simulink model "sampleModel1736"  (R2022a)
settings: Solver=FixedStepAuto  StartTime=0.0  StopTime=10.0  RelTol=1e-3
undefined symbols (not defined in the file): DiscIntNeverNeededParam, magnitude, Newton, Raphson
libraries: simulink x102, slpidlib x27
(part 1 of 4)
settings Model: SimulationMode=software-in-the-loop (sil)  Creator=lenovo  LastModifiedBy=TSMC
settings DataIOCC: InspectSignalLogs=on  SignalLoggingName=logsOut
settings OptimizationCC: DefaultParameterBehavior=Inlined  EnhancedBackFolding=on  PassReuseOutputArgsAs=Individual arguments  ZeroExternalMemoryAtStartup=off  ZeroInternalMemoryAtStartup=off  OptimizeBlockOrder=speed  DifferentSizesBufferReuse=on  OptimizationCustomize=off  EfficientTunableParamExpr=on
settings DebuggingCC: ParameterTunabilityLossMsg=error  UnconnectedInputMsg=warning  UnconnectedOutputMsg=warning  UnconnectedLineMsg=warning
settings ModelReferenceCC: UpdateModelReferenceTargets=Force
settings SFSimCC: MATLABDynamicMemAlloc=off
settings RTWCC: SystemTargetFile=ert.tlc  TemplateMakefile=ert_default_tmf  GenerateReport=on  IncludeHyperlinkInReport=on  GenerateTraceInfo=on  DLArmComputeVersion=19.05
settings CodeAppCC: ForceParamTrailComments=on  IgnoreCustomStorageClasses=off  OperatorAnnotations=on  SimulinkDataObjDesc=on  SFDataObjDesc=on  InsertBlockDesc=on
settings ERTTargetCC: TargetLangStandard=C99 (ISO)  GenerateSampleERTMain=on  SupportContinuousTime=on  InlinedParameterPlacement=NonHierarchical  ERTCustomFileTemplate=example_file_process.tlc

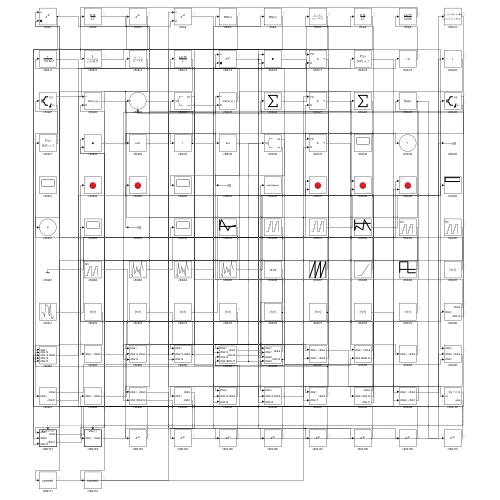
[thumbnail: Simulink's stored preview of the top-level diagram]
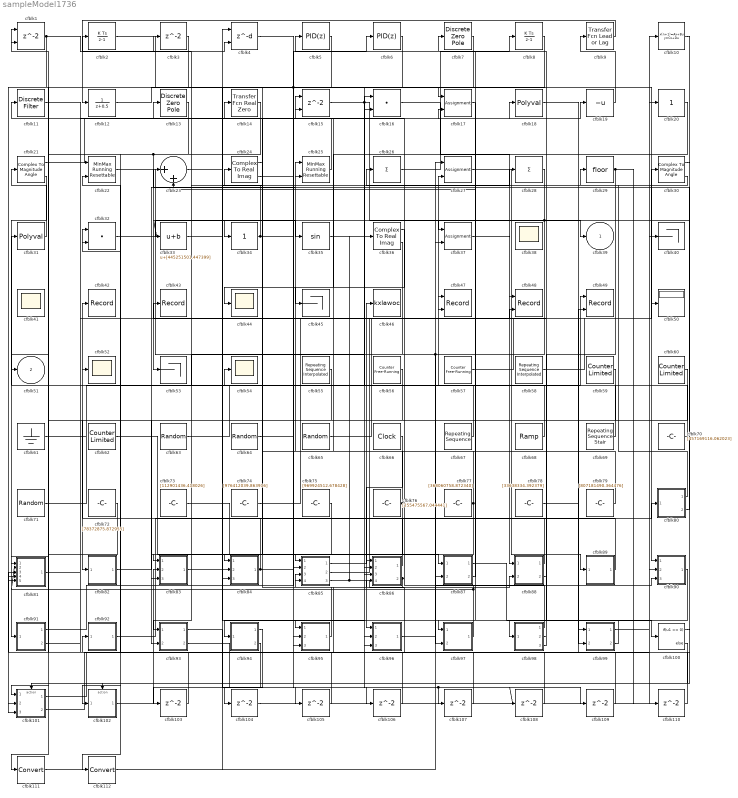
== system sampleModel1736 ==
  cfblk1 : Delay  ShowEnablePort=on  SampleTime=1
      settings: InputPortMap=u0,e6
  cfblk10 : DiscreteStateSpace
  cfblk100 : If  IfExpression=u1 >= 0  SampleTime=1
  cfblk101 : Subsystem  TreatAsAtomicUnit=on
  cfblk102 : Subsystem  TreatAsAtomicUnit=on
  cfblk{3,103..110} (9 alike) : Delay  SampleTime=1
  cfblk11 : DiscreteFilter  SampleTime=1
  cfblk111 : DataTypeConversion  SaturateOnIntegerOverflow=off  RndMeth=Floor
  cfblk112 : DataTypeConversion  SaturateOnIntegerOverflow=off  RndMeth=Floor
  cfblk12 : DiscreteTransferFcn  SampleTime=1
  cfblk13 : DiscreteZeroPole  Poles=[0 0.5]  Gain=1
  cfblk14 : simulink/Discrete/Transfer Fcn Real Zero  ZeroZ=0.75  ICPrevInput=0.0  DoSatur=off
      settings: SourceProductBaseCode=SL
  cfblk15 : Delay  ShowEnablePort=on  SampleTime=1
      settings: InputPortMap=u0,e6
  cfblk16 : DotProduct  OutDataTypeStr=Inherit: Inherit via internal rule
  cfblk17 : Assignment  DiagnosticForDimensions=Warning  IndexOptions=Index vector (dialog)  Indices=1  OutputSizes=1
  cfblk18 : Polyval  Coefs=[ +2.081618890e-019, -1.441693666e-014, +4.719686976e-010, -8.536869453e-006, +1.621573104e-001, -8.087801117e+001 ]
  cfblk19 : UnaryMinus
  cfblk2 : DiscreteIntegrator  ICPrevOutput=DiscIntNeverNeededParam  ICPrevScaledInput=DiscIntNeverNeededParam
  cfblk20 : simulink/Math Operations/Slider Gain  gain=1  low=0  high=2
  cfblk21 : ComplexToMagnitudeAngle
  cfblk22 : simulink/Math Operations/MinMax Running Resettable  Function=min  vinit=0.0
  cfblk23 : Sum  Inputs=|++
  cfblk24 : ComplexToRealImag
  cfblk25 : simulink/Math Operations/MinMax Running Resettable  Function=min  vinit=0.0
  cfblk26 : Sum  Inputs=+
  cfblk27 : Assignment  DiagnosticForDimensions=Warning  IndexOptions=Index vector (dialog)  Indices=1  OutputSizes=1
  cfblk28 : Sum  Inputs=+
  cfblk29 : Rounding
  cfblk30 : ComplexToMagnitudeAngle
  cfblk31 : Polyval  Coefs=[ +2.081618890e-019, -1.441693666e-014, +4.719686976e-010, -8.536869453e-006, +1.621573104e-001, -8.087801117e+001 ]
  cfblk32 : DotProduct  OutDataTypeStr=Inherit: Inherit via internal rule
  cfblk33 : Bias  Bias=[445251501.447399]  SaturateOnIntegerOverflow=off
  cfblk34 : simulink/Math Operations/Slider Gain  gain=1  low=0  high=2
  cfblk35 : Trigonometry
  cfblk36 : ComplexToRealImag
  cfblk37 : Assignment  DiagnosticForDimensions=Warning  IndexOptions=Index vector (dialog)  Indices=1  OutputSizes=1
  cfblk{38,41,44,52,54} (5 alike) : Scope
      cfblk38 settings: Floating=on
      cfblk41 settings: Floating=on
  cfblk4 : Delay  DelayLengthSource=Input port  SampleTime=1
      settings: InputPortMap=u0,p1
  cfblk40 : Terminator
  cfblk42 : Record  FileSettingsInternal="{\"entries\":[{\"content\":{\"excelSettings\":{\"content\":{},\"type\":\"Streamout.ExcelSettings\"}},\"type\":\"Streamout.FileSettingStorage\",\"uuid\":\"672957eb-ee49-4fe5-a35a-1dea1006cdd7\"}],\"packageUris\":[\"http://schema.mathworks.com/mf0/streamout_blocks/R2020a\"],\"version\":\"1.0\"}"  SignalsInternal="{\"entries\":[{\"content\":{\"signals\":[]},\"type\":\"RecordBlkView.InputSignals\",\"uuid\":\"5e46232b-0d34-4261-b03a-cdc6809bb342\"}],\"packageUris\":[\"http://schema.mathworks.com/mf0/streamout_blocks/R2020a\"],\"version\":\"1.0\"}"  VisualizationBindings="{\"sparklinesplugin\":{\"info\":[{\"bindingParametersList\":[],\"subplotID\":1}]}}"
  cfblk43 : Record  FileSettingsInternal="{\"entries\":[{\"content\":{\"excelSettings\":{\"content\":{},\"type\":\"Streamout.ExcelSettings\"}},\"type\":\"Streamout.FileSettingStorage\",\"uuid\":\"393a2e3c-94c8-4af6-8f54-ad1e74355c79\"}],\"packageUris\":[\"http://schema.mathworks.com/mf0/streamout_blocks/R2020a\"],\"version\":\"1.0\"}"  SignalsInternal="{\"entries\":[{\"content\":{\"signals\":[]},\"type\":\"RecordBlkView.InputSignals\",\"uuid\":\"d289a954-6309-4463-a7cf-1981229a1c79\"}],\"packageUris\":[\"http://schema.mathworks.com/mf0/streamout_blocks/R2020a\"],\"version\":\"1.0\"}"  VisualizationBindings="{\"sparklinesplugin\":{\"info\":[{\"bindingParametersList\":[],\"subplotID\":1}]}}"
  cfblk45 : Terminator
  cfblk46 : ToWorkspace  VariableName=kxlawoc  SaveFormat=Timeseries  SampleTime=-1
  cfblk47 : Record  FileSettingsInternal="{\"entries\":[{\"content\":{\"excelSettings\":{\"content\":{},\"type\":\"Streamout.ExcelSettings\"}},\"type\":\"Streamout.FileSettingStorage\",\"uuid\":\"0105e05e-0964-4cfc-9bef-5427dfc10fd6\"}],\"packageUris\":[\"http://schema.mathworks.com/mf0/streamout_blocks/R2020a\"],\"version\":\"1.0\"}"  Layout=[1 1]  SignalsInternal="{\"entries\":[{\"content\":{\"signals\":[]},\"type\":\"RecordBlkView.InputSignals\",\"uuid\":\"b76d1c99-58a2-4a2f-b9d3-63975c932613\"}],\"packageUris\":[\"http://schema.mathworks.com/mf0/streamout_blocks/R2020a\"],\"version\":\"1.0\"}"  VisualizationBindings="{\"xyplotplugin\":{\"info\":[{\"series\":[],\"subplotID\":1}]}}"  CompatibilityTag=XY  st=-1
  cfblk48 : Record  FileSettingsInternal="{\"entries\":[{\"content\":{\"excelSettings\":{\"content\":{},\"type\":\"Streamout.ExcelSettings\"}},\"type\":\"Streamout.FileSettingStorage\",\"uuid\":\"b0e192a8-91e4-4ef8-ad00-b270703470c1\"}],\"packageUris\":[\"http://schema.mathworks.com/mf0/streamout_blocks/R2020a\"],\"version\":\"1.0\"}"  Layout=[1 1]  SignalsInternal="{\"entries\":[{\"content\":{\"signals\":[]},\"type\":\"RecordBlkView.InputSignals\",\"uuid\":\"d4c1af31-3cad-49f8-ac33-698687fb22b3\"}],\"packageUris\":[\"http://schema.mathworks.com/mf0/streamout_blocks/R2020a\"],\"version\":\"1.0\"}"  VisualizationBindings="{\"xyplotplugin\":{\"info\":[{\"series\":[],\"subplotID\":1}]}}"  CompatibilityTag=XY  st=-1
  cfblk49 : Record  FileSettingsInternal="{\"entries\":[{\"content\":{\"excelSettings\":{\"content\":{},\"type\":\"Streamout.ExcelSettings\"}},\"type\":\"Streamout.FileSettingStorage\",\"uuid\":\"edb0e36a-dec4-460e-bf37-95f7f6bcaa08\"}],\"packageUris\":[\"http://schema.mathworks.com/mf0/streamout_blocks/R2020a\"],\"version\":\"1.0\"}"  Layout=[1 1]  SignalsInternal="{\"entries\":[{\"content\":{\"signals\":[]},\"type\":\"RecordBlkView.InputSignals\",\"uuid\":\"dacf59fe-381c-43c7-bd7c-2111ca233486\"}],\"packageUris\":[\"http://schema.mathworks.com/mf0/streamout_blocks/R2020a\"],\"version\":\"1.0\"}"  VisualizationBindings="{\"xyplotplugin\":{\"info\":[{\"series\":[],\"subplotID\":1}]}}"  CompatibilityTag=XY  st=-1
  cfblk5 : slpidlib/PID Controller  Controller=PID  Form=Parallel  TimeDomain=Discrete-time  UseExternalTs=off  SampleTime=1  IntegratorMethod=Forward Euler  FilterMethod=Forward Euler  ControllerParametersSource=internal  P=1  I=1  UseKiTs=off  D=0  N=100  UseFilter=on  TunerSelectOption=Transfer Function Based (PID Tuner App)  InitialConditionSource=internal  InitialConditionForIntegrator=0  InitialConditionForFilter=0  DifferentiatorICPrevScaledInput=0  ExternalReset=none  TrackingMode=off  Kt=1  LimitOutput=off  SatLimitsSource=internal  UpperSaturationLimit=inf  LowerSaturationLimit=-inf  LinearizeAsGain=off  AntiWindupMode=none  Kb=1  POutMin=[]  POutMax=[]  IOutMin=[]  IOutMax=[]  DOutMin=[]  DOutMax=[]  NOutMin=[]  NOutMax=[]  SumOutMin=[]  SumOutMax=[]  SaturationOutMin=[]  SaturationOutMax=[]  PParamMin=[]  PParamMax=[]  IParamMin=[]  IParamMax=[]  DParamMin=[]  DParamMax=[]  NParamMin=[]  NParamMax=[]  KbParamMin=[]  KbParamMax=[]  KtParamMin=[]  KtParamMax=[]  KbOutMin=[]  KbOutMax=[]  KtOutMin=[]  KtOutMax=[]  IntegratorOutMin=[]  IntegratorOutMax=[]  FilterOutMin=[]  FilterOutMax=[]  SumI1OutMin=[]  SumI1OutMax=[]  SumI2OutMin=[]  SumI2OutMax=[]  SumI3OutMin=[]  SumI3OutMax=[]  SumI4OutMin=[]  SumI4OutMax=[]  SumDOutMin=[]  SumDOutMax=[]  DifferentiatorOutMin=[]  DifferentiatorOutMax=[]  FilterDiffOutCoefMin=[]  FilterDiffOutCoefMax=[]  ReciprocalOutMin=[]  ReciprocalOutMax=[]  SumDenOutMin=[]  SumDenOutMax=[]  SumNumOutMin=[]  SumNumOutMax=[]  DivideOutMin=[]  DivideOutMax=[]  UdiffTsProdOutMin=[]  UdiffTsProdOutMax=[]  NTsProdOutMin=[]  NTsProdOutMax=[]  UintegralTsProdOutMin=[]  UintegralTsProdOutMax=[]  UngainTsProdOutMin=[]  UngainTsProdOutMax=[]  IntegratorContinuousStateAttributes=''  IntegratorStateMustResolveToSignalObject=off  IntegratorRTWStateStorageClass=Auto  FilterContinuousStateAttributes=''  FilterStateMustResolveToSignalObject=off  FilterRTWStateStorageClass=Auto  ParallelPVariant=InternalParameters  IdealPVariant=Disabled  IVariant=InternalParameters  DVariant=InternalParameters  IntegratorVariant=Discrete  SatVariant=Disabled  AWVariant=Passthrough  PCopyVariant=Disabled  TRVariant=Disabled  FdbkBlocksVariant=Forward  IdealPFdbkVariant=Disabled  SatFdbkVariant=Disabled  DerivativeFilterVariant=ForwardEulerFilter  NVariant=InternalParameters  NCopyVariant=Disabled  FilterICVariant=InternalICsFilter  IntegratorICVariant=InternalICs  ExternalResetVariant=Disabled  TRSumVariant=Passthrough  SumFdbkVariant=Disabled  SumVariant=Sum_PID  TsampFilterVariant=InternalTs  TsampNgainVariant=Passthrough  TsampIntegralVariant=Passthrough  ExternalSaturationOutDataTypeStr=Inherit: Same as second input  aMode=0
  cfblk50 : Display
  cfblk53 : Terminator
  cfblk55 : simulink/Sources/Repeating Sequence Interpolated  OutValues=[104230047.262219, 599428898.796120, -374314563.310813, -77159658.418539, 103238874.330711]  TimeValues=[0 0.1 0.5 0.6 1].'  LookUpMeth=Use Input Nearest  tsamp=0.01  OutMin=[]  OutMax=[]  OutDataTypeStr=double  OutputDataTypeScalingMode=double  OutDataType=fixdt(0,8)  OutScaling=2^-10
  cfblk56 : simulink/Sources/Counter Free-Running  NumBits=[22.000000]  tsamp=-1
  cfblk57 : simulink/Sources/Counter Free-Running  NumBits=[57.000000]  tsamp=-1
  cfblk58 : simulink/Sources/Repeating Sequence Interpolated  OutValues=[-875191408.615631, -334490534.402374, -930210248.443409, 512312619.812677, -987378266.190417]  TimeValues=[0 0.1 0.5 0.6 1].'  LookUpMeth=Use Input Below  tsamp=0.01  OutMin=[]  OutMax=[]  OutDataTypeStr=double  OutputDataTypeScalingMode=double  OutDataType=fixdt(0,8)  OutScaling=2^-10
  cfblk59 : simulink/Sources/Counter Limited  uplimit=[368.000000]  tsamp=-1
  cfblk6 : slpidlib/PID Controller  Controller=PID  Form=Parallel  TimeDomain=Discrete-time  UseExternalTs=off  SampleTime=1  IntegratorMethod=Forward Euler  FilterMethod=Forward Euler  ControllerParametersSource=internal  P=1  I=1  UseKiTs=off  D=0  N=100  UseFilter=on  TunerSelectOption=Transfer Function Based (PID Tuner App)  InitialConditionSource=internal  InitialConditionForIntegrator=0  InitialConditionForFilter=0  DifferentiatorICPrevScaledInput=0  ExternalReset=none  TrackingMode=off  Kt=1  LimitOutput=off  SatLimitsSource=internal  UpperSaturationLimit=inf  LowerSaturationLimit=-inf  LinearizeAsGain=off  AntiWindupMode=none  Kb=1  POutMin=[]  POutMax=[]  IOutMin=[]  IOutMax=[]  DOutMin=[]  DOutMax=[]  NOutMin=[]  NOutMax=[]  SumOutMin=[]  SumOutMax=[]  SaturationOutMin=[]  SaturationOutMax=[]  PParamMin=[]  PParamMax=[]  IParamMin=[]  IParamMax=[]  DParamMin=[]  DParamMax=[]  NParamMin=[]  NParamMax=[]  KbParamMin=[]  KbParamMax=[]  KtParamMin=[]  KtParamMax=[]  KbOutMin=[]  KbOutMax=[]  KtOutMin=[]  KtOutMax=[]  IntegratorOutMin=[]  IntegratorOutMax=[]  FilterOutMin=[]  FilterOutMax=[]  SumI1OutMin=[]  SumI1OutMax=[]  SumI2OutMin=[]  SumI2OutMax=[]  SumI3OutMin=[]  SumI3OutMax=[]  SumI4OutMin=[]  SumI4OutMax=[]  SumDOutMin=[]  SumDOutMax=[]  DifferentiatorOutMin=[]  DifferentiatorOutMax=[]  FilterDiffOutCoefMin=[]  FilterDiffOutCoefMax=[]  ReciprocalOutMin=[]  ReciprocalOutMax=[]  SumDenOutMin=[]  SumDenOutMax=[]  SumNumOutMin=[]  SumNumOutMax=[]  DivideOutMin=[]  DivideOutMax=[]  UdiffTsProdOutMin=[]  UdiffTsProdOutMax=[]  NTsProdOutMin=[]  NTsProdOutMax=[]  UintegralTsProdOutMin=[]  UintegralTsProdOutMax=[]  UngainTsProdOutMin=[]  UngainTsProdOutMax=[]  IntegratorContinuousStateAttributes=''  IntegratorStateMustResolveToSignalObject=off  IntegratorRTWStateStorageClass=Auto  FilterContinuousStateAttributes=''  FilterStateMustResolveToSignalObject=off  FilterRTWStateStorageClass=Auto  ParallelPVariant=InternalParameters  IdealPVariant=Disabled  IVariant=InternalParameters  DVariant=InternalParameters  IntegratorVariant=Discrete  SatVariant=Disabled  AWVariant=Passthrough  PCopyVariant=Disabled  TRVariant=Disabled  FdbkBlocksVariant=Forward  IdealPFdbkVariant=Disabled  SatFdbkVariant=Disabled  DerivativeFilterVariant=ForwardEulerFilter  NVariant=InternalParameters  NCopyVariant=Disabled  FilterICVariant=InternalICsFilter  IntegratorICVariant=InternalICs  ExternalResetVariant=Disabled  TRSumVariant=Passthrough  SumFdbkVariant=Disabled  SumVariant=Sum_PID  TsampFilterVariant=InternalTs  TsampNgainVariant=Passthrough  TsampIntegralVariant=Passthrough  ExternalSaturationOutDataTypeStr=Inherit: Same as second input  aMode=0
  cfblk60 : simulink/Sources/Counter Limited  uplimit=[440.000000]  tsamp=-1
  cfblk61 : Ground
  cfblk62 : simulink/Sources/Counter Limited  uplimit=[704.000000]  tsamp=-1
  cfblk63 : UniformRandomNumber  Minimum=[-8414418817.122449]  Maximum=[8895670179.092813]  Seed=[31967642.000000]  SampleTime=0.1
  cfblk64 : UniformRandomNumber  Minimum=[-8128054304.758234]  Maximum=[2684039457.444082]  Seed=[42844118.000000]  SampleTime=0.1
  cfblk65 : UniformRandomNumber  Minimum=[-5959780952.881649]  Maximum=[115027929.744010]  Seed=[15221819.000000]  SampleTime=0.1
  cfblk66 : DigitalClock
  cfblk67 : simulink/Sources/Repeating Sequence  rep_seq_t=[0 2]  rep_seq_y=[-650847051.997155, 235497574.481386]
  cfblk68 : simulink/Sources/Ramp  slope=[2631.608105]  start=[23.947320]  InitialOutput=[-207313.322722]
  cfblk69 : simulink/Sources/Repeating Sequence Stair  OutValues=[147179978.901561, -65896230.958762]  tsamp=-1  OutMin=[]  OutMax=[]  OutDataTypeStr=double  OutputDataTypeScalingMode=double  OutDataType=fixdt(0,8)  ConRadixGroup=Best Precision: Vector-wise  OutScaling=2^-12
  cfblk7 : DiscreteZeroPole  Poles=[0 0.5]  Gain=1
  cfblk70 : Constant  Value=[457169116.062023]  SampleTime=1
  cfblk71 : RandomNumber  Mean=[51220.368146]  Variance=[79234.809419]  Seed=[59803815.000000]  SampleTime=0.1
  cfblk72 : Constant  Value=[78372875.872955]  SampleTime=1
  cfblk73 : Constant  Value=[112901436.418026]  SampleTime=1
  cfblk74 : Constant  Value=[976412039.863916]  SampleTime=1
  cfblk75 : Constant  Value=[969924512.678428]  SampleTime=1
  cfblk76 : Constant  Value=[255475567.044441]  SampleTime=1
  cfblk77 : Constant  Value=[368060758.872340]  SampleTime=1
  cfblk78 : Constant  Value=[33638334.392379]  SampleTime=1
  cfblk79 : Constant  Value=[807181490.364476]  SampleTime=1
  cfblk8 : DiscreteIntegrator  ICPrevOutput=DiscIntNeverNeededParam  ICPrevScaledInput=DiscIntNeverNeededParam
  cfblk80 : Subsystem
  cfblk81 : Subsystem
  cfblk82 : Subsystem
  cfblk83 : Subsystem
  cfblk84 : Subsystem
  cfblk85 : Subsystem
  cfblk86 : Subsystem
  cfblk87 : Subsystem
  cfblk88 : Subsystem
  cfblk89 : Subsystem
  cfblk9 : simulink/Discrete/Transfer Fcn Lead or Lag  PoleZ=0.95  ZeroZ=0.75  ICPrevOutput=0.0  ICPrevInput=0.0  DoSatur=off
      settings: SourceProductBaseCode=SL
  cfblk90 : Subsystem
  cfblk91 : Subsystem
  cfblk92 : Subsystem
  cfblk93 : Subsystem
  cfblk94 : Subsystem
  cfblk95 : Subsystem
  cfblk96 : Subsystem
  cfblk97 : Subsystem
  cfblk98 : Subsystem
  cfblk99 : Subsystem
  cfblk39 : Outport
  cfblk51 : Outport  Port=2
  wires:
  cfblk32/1 -> cfblk34/1
  cfblk21/1 -> cfblk13/1
  cfblk79/1 -> cfblk25/1
  cfblk95/1(cfblk2) -> cfblk24/1
  cfblk2/1 -> cfblk90/1(cfblk1)
  cfblk92/1(cfblk2) -> cfblk80/1(cfblk1)
  cfblk98/1(cfblk2) -> cfblk85/1(cfblk1)
  cfblk9/1 -> cfblk12/1
  cfblk10/1 -> cfblk92/1(cfblk1)
  cfblk71/1 -> cfblk49/1
  cfblk26/1 -> cfblk8/1
  cfblk75/1 -> cfblk83/1(cfblk1)
  cfblk66/1 -> cfblk96/1(cfblk1)
  cfblk76/1 -> cfblk14/1, cfblk95/2(cfblk15)
  cfblk25/1 -> cfblk11/1
  cfblk15/1 -> cfblk107/1, cfblk108/1, cfblk39/1
  cfblk27/1 -> cfblk89/1(cfblk1)
  cfblk23/1 -> cfblk96/2(cfblk15)
  cfblk85/1(cfblk2) -> cfblk46/1
  cfblk56/1 -> cfblk82/1(cfblk1)
  cfblk13/1 -> cfblk53/1, cfblk81/1(cfblk1)
  cfblk99/1(cfblk2) -> cfblk10/1
  cfblk37/1 -> cfblk88/1(cfblk1)
  cfblk102/1(cfblk2) -> cfblk83/2(cfblk13)
  cfblk85/2(cfblk16) -> cfblk30/1
  cfblk82/1(cfblk2) -> cfblk25/2
  cfblk21/2 -> cfblk91/1(cfblk1)
  cfblk80/1(cfblk2) -> cfblk29/1
  cfblk16/1 -> cfblk48/1
  cfblk85/3(cfblk17) -> cfblk88/2(cfblk13), cfblk36/1
  cfblk67/1 -> cfblk1/1
  cfblk5/1 -> cfblk84/1(cfblk1)
  cfblk65/1 -> cfblk27/2
  cfblk64/1 -> cfblk85/2(cfblk13)
  cfblk18/1 -> cfblk99/1(cfblk1)
  cfblk72/1 -> cfblk101/1(cfblk1)
  cfblk70/1 -> cfblk31/1
  cfblk31/1 -> cfblk21/1
  cfblk34/1 -> cfblk2/1, cfblk109/1
  cfblk97/1(cfblk2) -> cfblk54/1, cfblk81/2(cfblk12)
  cfblk89/1(cfblk2) -> cfblk42/1
  cfblk7/1 -> cfblk101/2(cfblk9), cfblk95/3(cfblk16)
  cfblk83/1(cfblk2) -> cfblk28/1
  cfblk20/1 -> cfblk45/1
  cfblk6/1 -> cfblk84/2(cfblk13)
  cfblk24/1 -> cfblk84/3(cfblk14)
  cfblk61/1 -> cfblk47/1
  cfblk98/2(cfblk16) -> cfblk5/1
  cfblk69/1 -> cfblk7/1
  cfblk88/1(cfblk2) -> cfblk22/2
  cfblk17/1 -> cfblk97/1(cfblk1)
  cfblk19/1 -> cfblk9/1
  cfblk96/1(cfblk2) -> cfblk90/3(cfblk7)
  cfblk30/1 -> cfblk37/1
  cfblk101/1(cfblk2) -> cfblk49/2
  cfblk58/1 -> cfblk50/1
  cfblk91/1(cfblk2) -> cfblk19/1
  cfblk91/2(cfblk11) -> cfblk48/2
  cfblk98/3(cfblk17) -> cfblk47/2
  cfblk68/1 -> cfblk3/1
  cfblk101/2(cfblk11) -> cfblk40/1
  cfblk77/1 -> cfblk83/3(cfblk14), cfblk15/1
  cfblk99/2(cfblk7) -> cfblk95/1(cfblk1)
  cfblk62/1 -> cfblk87/1(cfblk1)
  cfblk22/1 -> cfblk96/3(cfblk16)
  cfblk73/1 -> cfblk87/2(cfblk7)
  cfblk80/2(cfblk14) -> cfblk23/1
  cfblk14/1 -> cfblk102/1(cfblk1)
  cfblk81/1(cfblk2) -> cfblk18/1
  cfblk36/1 -> cfblk44/1
  cfblk24/2 -> cfblk6/1
  cfblk57/1 -> cfblk20/1
  cfblk36/2 -> cfblk93/1(cfblk1)
  cfblk84/1(cfblk2) -> cfblk86/1(cfblk1), cfblk32/1
  cfblk3/1 -> cfblk51/1
  cfblk8/1 -> cfblk101/3(cfblk10)
  cfblk28/1 -> cfblk97/2(cfblk17), cfblk86/3(cfblk8), cfblk33/1
  cfblk63/1 -> cfblk16/1
  cfblk30/2 -> cfblk26/1
  cfblk33/1 -> cfblk35/1
  cfblk55/1 -> cfblk93/2(cfblk11)
  cfblk87/1(cfblk2) -> cfblk100/1
  cfblk88/2(cfblk14) -> cfblk43/1
  cfblk87/2(cfblk8) -> cfblk23/2
  cfblk1/1 -> cfblk4/2, cfblk81/5(cfblk15)
  cfblk35/1 -> cfblk86/2(cfblk7)
  cfblk86/1(cfblk2) -> cfblk52/1
  cfblk4/1 -> cfblk16/2
  cfblk86/2(cfblk10) -> cfblk85/3(cfblk14), cfblk15/2
  cfblk74/1 -> cfblk37/2
  cfblk78/1 -> cfblk99/2(cfblk6)
  cfblk29/1 -> cfblk98/1(cfblk1), cfblk110/1
  cfblk12/1 -> cfblk17/1
  cfblk90/1(cfblk2) -> cfblk94/1(cfblk1)
  cfblk11/1 -> cfblk17/2
  cfblk100/1 -> cfblk101/Action
  cfblk100/2 -> cfblk102/Action
  cfblk94/1(cfblk2) -> cfblk103/1
  cfblk103/1 -> cfblk22/1
  cfblk94/2(cfblk7) -> cfblk104/1
  cfblk104/1 -> cfblk90/2(cfblk6)
  cfblk93/1(cfblk2) -> cfblk105/1
  cfblk105/1 -> cfblk1/2
  cfblk93/2(cfblk12) -> cfblk106/1
  cfblk106/1 -> cfblk85/4(cfblk15)
  cfblk107/1 -> cfblk81/4(cfblk14)
  cfblk108/1 -> cfblk86/4(cfblk9)
  cfblk109/1 -> cfblk32/2
  cfblk110/1 -> cfblk81/3(cfblk13)
  cfblk60/1 -> cfblk111/1
  cfblk111/1 -> cfblk27/1
  cfblk59/1 -> cfblk112/1
  cfblk112/1 -> cfblk4/1

== system sampleModel1736/cfblk101 ==
  cfblk1 : Inport
  cfblk9 : Inport  Port=2
  cfblk10 : Inport  Port=3
  Action Port : ActionPort  ActionPortLabel=if(u1 >= 0)
  cfblk12 : Delay
  cfblk13 : Delay
  cfblk14 : Delay
  cfblk3 : Delay  ShowEnablePort=on
      settings: InputPortMap=u0,e6
  cfblk4 : Sum  Inputs=+-
  cfblk5 : Reshape
  cfblk6 : Product
  cfblk7 : Product  Inputs=*
  cfblk8 : Subsystem
  cfblk2 : Outport
  cfblk11 : Outport  Port=2
  wires:
  cfblk5/1 -> cfblk2/1
  cfblk7/1 -> cfblk11/1
  cfblk3/1 -> cfblk7/1, cfblk13/1
  cfblk1/1 -> cfblk8/2(cfblk13), cfblk5/1
  cfblk10/1 -> cfblk6/1, cfblk4/2
  cfblk9/1 -> cfblk3/1
  cfblk8/1(cfblk2) -> cfblk4/1
  cfblk8/2(cfblk16) -> cfblk3/2, cfblk6/2
  cfblk4/1 -> cfblk12/1
  cfblk12/1 -> cfblk8/1(cfblk1)
  cfblk13/1 -> cfblk8/4(cfblk15)
  cfblk6/1 -> cfblk14/1
  cfblk14/1 -> cfblk8/3(cfblk14)

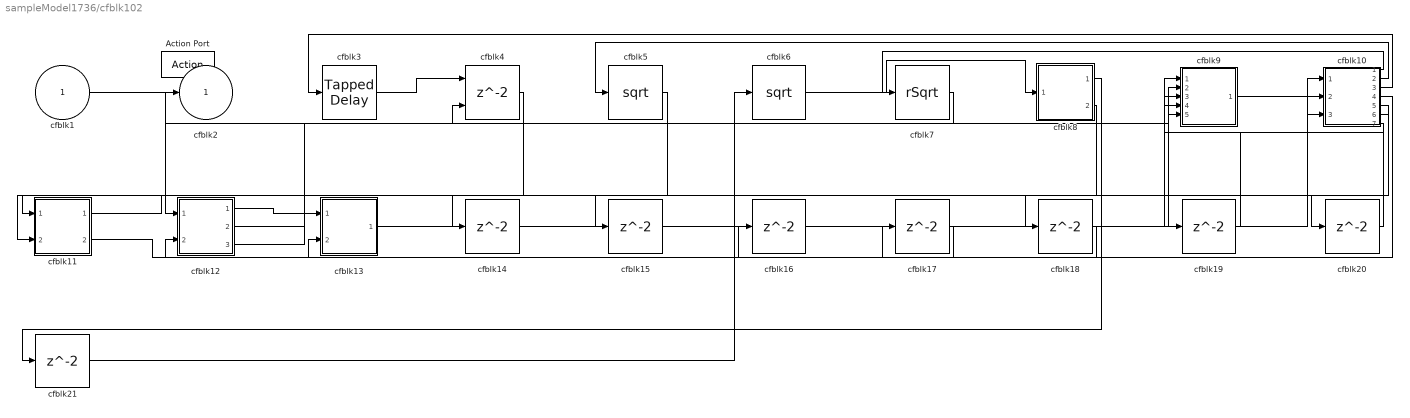
== system sampleModel1736/cfblk102 ==
  cfblk1 : Inport
  Action Port : ActionPort  ActionPortLabel=else
  cfblk10 : Subsystem
  cfblk11 : Subsystem
  cfblk12 : Subsystem
  cfblk13 : Subsystem
  cfblk{14..21} (8 alike) : Delay
  cfblk3 : simulink/Discrete/Tapped Delay  vinit=0.0  samptime=-1  NumDelays=1  DelayOrder=Oldest  includeCurrent=off
  cfblk4 : Delay  ShowEnablePort=on
      settings: InputPortMap=u0,e6
  cfblk5 : Sqrt
  cfblk6 : Sqrt
  cfblk7 : Sqrt  Operator=rSqrt  AlgorithmType=Newton-Raphson
  cfblk8 : Subsystem
  cfblk9 : Subsystem
  cfblk2 : Outport
  wires:
  cfblk6/1 -> cfblk8/1(cfblk1)
  cfblk10/1(cfblk2) -> cfblk7/1
  cfblk4/1 -> cfblk11/1(cfblk1)
  cfblk8/2(cfblk10) -> cfblk11/2(cfblk6)
  cfblk1/1 -> cfblk12/1(cfblk1)
  cfblk10/2(cfblk11) -> cfblk5/1
  cfblk10/3(cfblk12) -> cfblk3/1
  cfblk13/1(cfblk2) -> cfblk9/2(cfblk11)
  cfblk12/1(cfblk2) -> cfblk13/1(cfblk1)
  cfblk7/1 -> cfblk2/1
  cfblk3/1 -> cfblk4/1
  cfblk9/1(cfblk2) -> cfblk10/3(cfblk10)
  cfblk12/2(cfblk9) -> cfblk4/2
  cfblk12/3(cfblk10) -> cfblk9/5(cfblk14)
  cfblk5/1 -> cfblk14/1
  cfblk14/1 -> cfblk10/1(cfblk1)
  cfblk11/1(cfblk2) -> cfblk15/1
  cfblk15/1 -> cfblk9/1(cfblk1)
  cfblk11/2(cfblk7) -> cfblk16/1
  cfblk16/1 -> cfblk10/2(cfblk9)
  cfblk10/4(cfblk13) -> cfblk17/1
  cfblk17/1 -> cfblk13/2(cfblk10)
  cfblk10/5(cfblk14) -> cfblk18/1
  cfblk18/1 -> cfblk12/2(cfblk8)
  cfblk10/6(cfblk15) -> cfblk19/1
  cfblk19/1 -> cfblk9/3(cfblk12)
  cfblk10/7(cfblk16) -> cfblk20/1
  cfblk20/1 -> cfblk9/4(cfblk13)
  cfblk8/1(cfblk2) -> cfblk21/1
  cfblk21/1 -> cfblk6/1

== system sampleModel1736/cfblk80 ==
  cfblk1 : Inport
  cfblk10 : Subsystem
  cfblk11 : Subsystem
  cfblk12 : Subsystem
  cfblk13 : Subsystem
  cfblk{15..18} (4 alike) : Delay  SampleTime=1
  cfblk3 : Delay  DelayLengthSource=Input port  SampleTime=1
      settings: InputPortMap=u0,p1
  cfblk4 : DiscreteIntegrator  ICPrevOutput=DiscIntNeverNeededParam  ICPrevScaledInput=DiscIntNeverNeededParam
  cfblk5 : Trigonometry
  cfblk6 : Constant  Value=[-55561184.217623]  SampleTime=1
  cfblk7 : Constant  Value=[-741018626.841991]  SampleTime=1
  cfblk8 : Constant  Value=[-397496421.896853]  SampleTime=1
  cfblk9 : Subsystem
  cfblk2 : Outport
  cfblk14 : Outport  Port=2
  wires:
  cfblk6/1 -> cfblk12/1(cfblk1)
  cfblk3/1 -> cfblk10/1(cfblk1)
  cfblk13/1(cfblk2) -> cfblk4/1
  cfblk7/1 -> cfblk11/1(cfblk1)
  cfblk8/1 -> cfblk10/3(cfblk13)
  cfblk12/1(cfblk2) -> cfblk3/2
  cfblk1/1 -> cfblk12/2(cfblk16)
  cfblk11/1(cfblk2) -> cfblk9/1(cfblk1)
  cfblk11/2(cfblk13) -> cfblk5/1
  cfblk4/1 -> cfblk2/1, cfblk16/1
  cfblk5/1 -> cfblk9/2(cfblk8)
  cfblk10/1(cfblk2) -> cfblk11/2(cfblk10)
  cfblk13/4(cfblk7) -> cfblk14/1
  cfblk10/2(cfblk16) -> cfblk11/3(cfblk11)
  cfblk10/3(cfblk17) -> cfblk11/4(cfblk12), cfblk13/1(cfblk1)
  cfblk9/1(cfblk2) -> cfblk15/1
  cfblk15/1 -> cfblk3/1
  cfblk16/1 -> cfblk10/4(cfblk14)
  cfblk13/2(cfblk5) -> cfblk17/1
  cfblk17/1 -> cfblk10/2(cfblk12)
  cfblk13/3(cfblk6) -> cfblk18/1
  cfblk18/1 -> cfblk10/5(cfblk15)

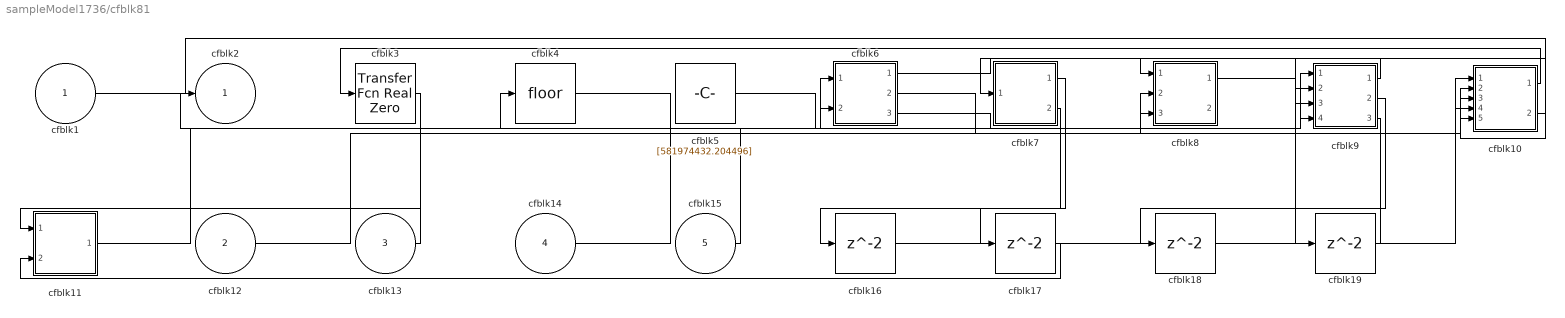
== system sampleModel1736/cfblk81 ==
  cfblk1 : Inport
  cfblk12 : Inport  Port=2
  cfblk13 : Inport  Port=3
  cfblk14 : Inport  Port=4
  cfblk15 : Inport  Port=5
  cfblk10 : Subsystem
  cfblk11 : Subsystem
  cfblk{16..19} (4 alike) : Delay  SampleTime=1
  cfblk3 : simulink/Discrete/Transfer Fcn Real Zero  ZeroZ=0.75  ICPrevInput=0.0  DoSatur=off
      settings: SourceProductBaseCode=SL
  cfblk4 : Rounding
  cfblk5 : Constant  Value=[581974432.204496]  SampleTime=1
  cfblk6 : Subsystem
  cfblk7 : Subsystem
  cfblk8 : Subsystem
  cfblk9 : Subsystem
  cfblk2 : Outport
  wires:
  cfblk11/1(cfblk2) -> cfblk9/1(cfblk1)
  cfblk9/1(cfblk2) -> cfblk7/1(cfblk1)
  cfblk10/1(cfblk2) -> cfblk3/1
  cfblk15/1 -> cfblk4/1
  cfblk14/1 -> cfblk6/1(cfblk1)
  cfblk1/1 -> cfblk10/2(cfblk13)
  cfblk12/1 -> cfblk10/3(cfblk14)
  cfblk6/1(cfblk2) -> cfblk9/2(cfblk12)
  cfblk3/1 -> cfblk11/1(cfblk1)
  cfblk10/2(cfblk17) -> cfblk8/1(cfblk1)
  cfblk9/3(cfblk16) -> cfblk8/2(cfblk12)
  cfblk4/1 -> cfblk6/2(cfblk9)
  cfblk5/1 -> cfblk8/3(cfblk13)
  cfblk6/2(cfblk10) -> cfblk10/5(cfblk16)
  cfblk13/1 -> cfblk2/1
  cfblk6/3(cfblk11) -> cfblk9/4(cfblk14)
  cfblk7/1(cfblk2) -> cfblk16/1
  cfblk16/1 -> cfblk10/1(cfblk1)
  cfblk7/2(cfblk9) -> cfblk17/1
  cfblk17/1 -> cfblk11/2(cfblk12)
  cfblk9/2(cfblk15) -> cfblk18/1
  cfblk18/1 -> cfblk10/4(cfblk15)
  cfblk8/1(cfblk2) -> cfblk19/1
  cfblk19/1 -> cfblk9/3(cfblk13)

== system sampleModel1736/cfblk82 ==
  cfblk1 : Inport
  cfblk3 : simulink/Discrete/Transfer Fcn Real Zero  ZeroZ=0.75  ICPrevInput=0.0  DoSatur=off
      settings: SourceProductBaseCode=SL
  cfblk4 : simulink/Discrete/Transfer Fcn First Order  PoleZ=0.95  ICPrevOutput=0.0  DoSatur=off
  cfblk5 : DiscreteFir  SampleTime=1
  cfblk6 : Bias  Bias=[569456576.995668]  SaturateOnIntegerOverflow=off
  cfblk7 : Subsystem
  cfblk8 : Delay  SampleTime=1
  cfblk2 : Outport
  wires:
  cfblk1/1 -> cfblk3/1
  cfblk4/1 -> cfblk6/1, cfblk5/1
  cfblk3/1 -> cfblk2/1
  cfblk5/1 -> cfblk7/1(cfblk1)
  cfblk6/1 -> cfblk7/2(cfblk10), cfblk7/3(cfblk11)
  cfblk7/1(cfblk2) -> cfblk8/1
  cfblk8/1 -> cfblk4/1

== system sampleModel1736/cfblk83 ==
  cfblk1 : Inport
  cfblk13 : Inport  Port=2
  cfblk14 : Inport  Port=3
  cfblk10 : Subsystem
  cfblk11 : Subsystem
  cfblk12 : Subsystem
  cfblk15 : Delay  SampleTime=1
  cfblk16 : Delay  SampleTime=1
  cfblk17 : Delay  SampleTime=1
  cfblk3 : simulink/Discrete/Transfer Fcn Real Zero  ZeroZ=0.75  ICPrevInput=0.0  DoSatur=off
      settings: SourceProductBaseCode=SL
  cfblk4 : Delay  DelayLengthSource=Input port  SampleTime=1
      settings: InputPortMap=u0,p1
  cfblk5 : Delay  DelayLengthSource=Input port  SampleTime=1
      settings: InputPortMap=u0,p1
  cfblk6 : DotProduct  OutDataTypeStr=Inherit: Inherit via internal rule
  cfblk7 : Product  Inputs=*
  cfblk8 : Sum  Inputs=+-
  cfblk9 : Subsystem
  cfblk2 : Outport
  wires:
  cfblk1/1 -> cfblk2/1
  cfblk13/1 -> cfblk3/1
  cfblk10/1(cfblk2) -> cfblk6/1
  cfblk8/1 -> cfblk9/1(cfblk1)
  cfblk4/1 -> cfblk5/2, cfblk10/2(cfblk8)
  cfblk5/1 -> cfblk8/1
  cfblk3/1 -> cfblk4/1, cfblk9/4(cfblk12)
  cfblk11/1(cfblk2) -> cfblk10/1(cfblk1)
  cfblk10/2(cfblk9) -> cfblk7/1
  cfblk12/2(cfblk15) -> cfblk6/2
  cfblk10/3(cfblk10) -> cfblk12/1(cfblk1)
  cfblk14/1 -> cfblk11/1(cfblk1), cfblk9/3(cfblk11)
  cfblk10/4(cfblk11) -> cfblk8/2
  cfblk9/1(cfblk2) -> cfblk12/2(cfblk12)
  cfblk7/1 -> cfblk12/3(cfblk13)
  cfblk9/2(cfblk13) -> cfblk12/4(cfblk14)
  cfblk12/1(cfblk2) -> cfblk15/1
  cfblk15/1 -> cfblk4/2
  cfblk6/1 -> cfblk16/1
  cfblk16/1 -> cfblk5/1
  cfblk12/3(cfblk16) -> cfblk17/1
  cfblk17/1 -> cfblk9/2(cfblk10)

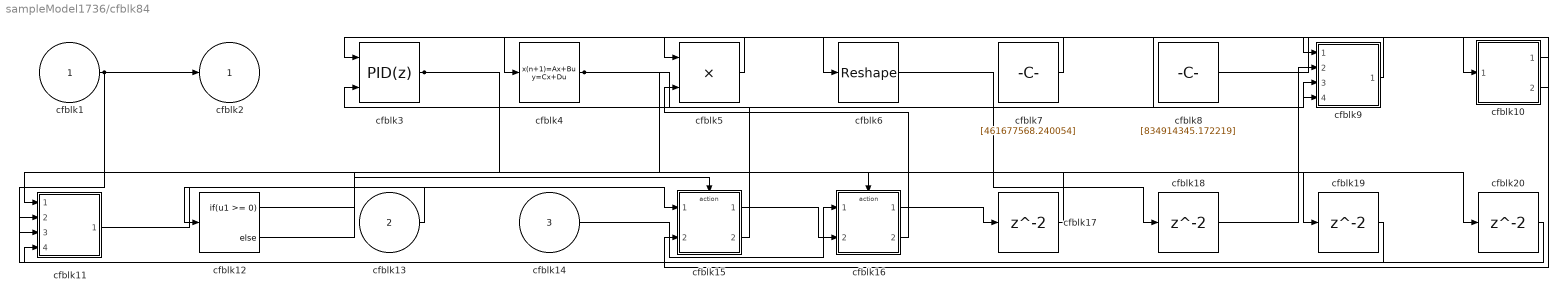
== system sampleModel1736/cfblk84 ==
  cfblk1 : Inport
  cfblk13 : Inport  Port=2
  cfblk14 : Inport  Port=3
  cfblk10 : Subsystem
  cfblk11 : Subsystem
  cfblk12 : If  IfExpression=u1 >= 0  SampleTime=1
  cfblk15 : Subsystem  TreatAsAtomicUnit=on
  cfblk16 : Subsystem  TreatAsAtomicUnit=on
  cfblk{17..20} (4 alike) : Delay  SampleTime=1
  cfblk3 : slpidlib/PID Controller (2DOF)  Controller=PID  Form=Parallel  TimeDomain=Discrete-time  UseExternalTs=off  SampleTime=1  IntegratorMethod=Forward Euler  FilterMethod=Forward Euler  ControllerParametersSource=internal  P=1  I=1  UseKiTs=off  D=0  N=100  UseFilter=on  b=1  c=1  TunerSelectOption=Transfer Function Based (PID Tuner App)  InitialConditionSource=internal  InitialConditionForIntegrator=0  InitialConditionForFilter=0  DifferentiatorICPrevScaledInput=0  ExternalReset=none  TrackingMode=off  Kt=1  LimitOutput=off  SatLimitsSource=internal  UpperSaturationLimit=inf  LowerSaturationLimit=-inf  LinearizeAsGain=off  AntiWindupMode=none  Kb=1  POutMin=[]  POutMax=[]  IOutMin=[]  IOutMax=[]  DOutMin=[]  DOutMax=[]  NOutMin=[]  NOutMax=[]  bOutMin=[]  bOutMax=[]  cOutMin=[]  cOutMax=[]  SumOutMin=[]  SumOutMax=[]  SaturationOutMin=[]  SaturationOutMax=[]  PParamMin=[]  PParamMax=[]  IParamMin=[]  IParamMax=[]  DParamMin=[]  DParamMax=[]  NParamMin=[]  NParamMax=[]  bParamMin=[]  bParamMax=[]  cParamMin=[]  cParamMax=[]  KbParamMin=[]  KbParamMax=[]  KtParamMin=[]  KtParamMax=[]  KbOutMin=[]  KbOutMax=[]  KtOutMin=[]  KtOutMax=[]  IntegratorOutMin=[]  IntegratorOutMax=[]  FilterOutMin=[]  FilterOutMax=[]  SumI1OutMin=[]  SumI1OutMax=[]  SumI2OutMin=[]  SumI2OutMax=[]  SumI3OutMin=[]  SumI3OutMax=[]  SumI4OutMin=[]  SumI4OutMax=[]  SumDOutMin=[]  SumDOutMax=[]  Sum1OutMin=[]  Sum1OutMax=[]  Sum2OutMin=[]  Sum2OutMax=[]  Sum3OutMin=[]  Sum3OutMax=[]  DifferentiatorOutMin=[]  DifferentiatorOutMax=[]  FilterDiffOutCoefMin=[]  FilterDiffOutCoefMax=[]  ReciprocalOutMin=[]  ReciprocalOutMax=[]  SumDenOutMin=[]  SumDenOutMax=[]  SumNumOutMin=[]  SumNumOutMax=[]  DivideOutMin=[]  DivideOutMax=[]  UdiffTsProdOutMin=[]  UdiffTsProdOutMax=[]  NTsProdOutMin=[]  NTsProdOutMax=[]  UintegralTsProdOutMin=[]  UintegralTsProdOutMax=[]  UngainTsProdOutMin=[]  UngainTsProdOutMax=[]  IntegratorContinuousStateAttributes=''  IntegratorStateMustResolveToSignalObject=off  IntegratorRTWStateStorageClass=Auto  FilterContinuousStateAttributes=''  FilterStateMustResolveToSignalObject=off  FilterRTWStateStorageClass=Auto  ParallelPVariant=InternalParameters  IdealPVariant=Disabled  IVariant=InternalParameters  DVariant=InternalParameters  bVariant=InternalParameters  cVariant=InternalParameters  IntegratorVariant=Discrete  SatVariant=Disabled  AWVariant=Passthrough  PCopyVariant=Disabled  TRVariant=Disabled  FdbkBlocksVariant=Forward  IdealPFdbkVariant=Disabled  SatFdbkVariant=Disabled  DerivativeFilterVariant=ForwardEulerFilter  NVariant=InternalParameters  NCopyVariant=Disabled  FilterICVariant=InternalICsFilter  IntegratorICVariant=InternalICs  ExternalResetVariant=Disabled  TRSumVariant=Passthrough  SumFdbkVariant=Disabled  SumVariant=Sum_PID  TsampFilterVariant=InternalTs  TsampNgainVariant=Passthrough  TsampIntegralVariant=Passthrough  ExternalSaturationOutDataTypeStr=Inherit: Same as second input
      settings: SourceProductBaseCode=SL
  cfblk4 : DiscreteStateSpace
  cfblk5 : Product
  cfblk6 : Reshape
  cfblk7 : Constant  Value=[461677568.240054]  SampleTime=1
  cfblk8 : Constant  Value=[834914345.172219]  SampleTime=1
  cfblk9 : Subsystem
  cfblk2 : Outport
  wires:
  cfblk11/1(cfblk2) -> cfblk15/1(cfblk1)
  cfblk5/1 -> cfblk4/1
  cfblk8/1 -> cfblk10/1(cfblk1)
  cfblk1/1 -> cfblk2/1, cfblk11/3(cfblk9)
  cfblk14/1 -> cfblk16/1(cfblk1)
  cfblk4/1 -> cfblk9/1(cfblk1), cfblk9/4(cfblk14), cfblk19/1
  cfblk9/1(cfblk2) -> cfblk6/1
  cfblk10/1(cfblk2) -> cfblk15/2(cfblk14)
  cfblk13/1 -> cfblk12/1
  cfblk7/1 -> cfblk5/1
  cfblk16/2(cfblk10) -> cfblk5/2
  cfblk15/1(cfblk2) -> cfblk16/2(cfblk9)
  cfblk10/2(cfblk8) -> cfblk3/1
  cfblk15/2(cfblk15) -> cfblk3/2
  cfblk3/1 -> cfblk9/3(cfblk13), cfblk20/1
  cfblk12/1 -> cfblk15/Action
  cfblk12/2 -> cfblk16/Action
  cfblk16/1(cfblk2) -> cfblk17/1
  cfblk17/1 -> cfblk11/1(cfblk1)
  cfblk6/1 -> cfblk18/1
  cfblk18/1 -> cfblk9/2(cfblk12)
  cfblk19/1 -> cfblk11/4(cfblk10)
  cfblk20/1 -> cfblk11/2(cfblk8)

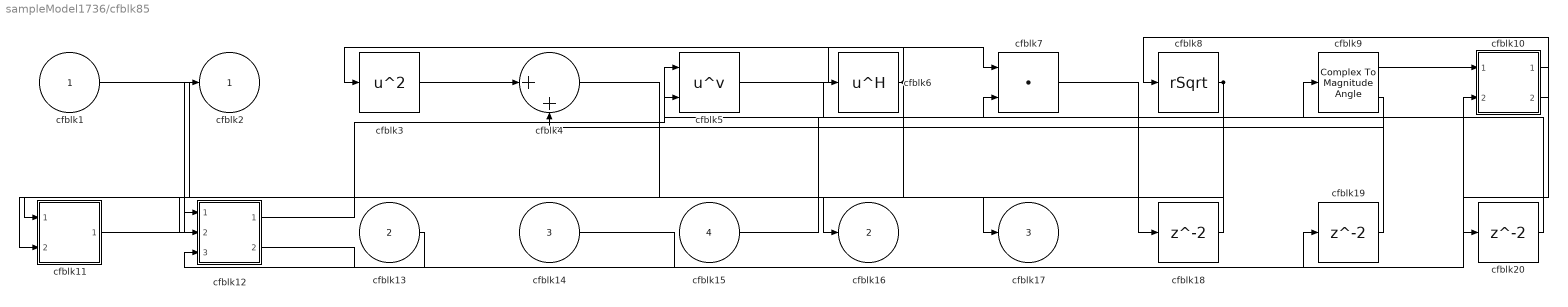
== system sampleModel1736/cfblk85 ==
  cfblk1 : Inport
  cfblk13 : Inport  Port=2
  cfblk14 : Inport  Port=3
  cfblk15 : Inport  Port=4
  cfblk10 : Subsystem
  cfblk11 : Subsystem
  cfblk12 : Subsystem
  cfblk18 : Delay  SampleTime=1
  cfblk19 : Delay  SampleTime=1
  cfblk20 : Delay  SampleTime=1
  cfblk3 : Math  Operator=square
  cfblk4 : Sum  Inputs=|++
  cfblk5 : Math  Operator=pow
  cfblk6 : Math  Operator=hermitian
  cfblk7 : DotProduct  OutDataTypeStr=Inherit: Inherit via internal rule
  cfblk8 : Sqrt  Operator=rSqrt  AlgorithmType=Newton-Raphson
  cfblk9 : ComplexToMagnitudeAngle
  cfblk2 : Outport
  cfblk16 : Outport  Port=2
  cfblk17 : Outport  Port=3
  wires:
  cfblk1/1 -> cfblk16/1
  cfblk11/1(cfblk2) -> cfblk2/1
  cfblk12/1(cfblk2) -> cfblk5/1
  cfblk8/1 -> cfblk12/1(cfblk1), cfblk11/2(cfblk8)
  cfblk5/1 -> cfblk7/1
  cfblk6/1 -> cfblk12/2(cfblk11), cfblk3/1, cfblk11/1(cfblk1)
  cfblk13/1 -> cfblk12/3(cfblk12)
  cfblk10/2(cfblk11) -> cfblk8/1
  cfblk9/1 -> cfblk10/1(cfblk1)
  cfblk3/1 -> cfblk4/1
  cfblk14/1 -> cfblk10/2(cfblk10)
  cfblk9/2 -> cfblk4/2
  cfblk15/1 -> cfblk7/2
  cfblk4/1 -> cfblk17/1
  cfblk7/1 -> cfblk18/1
  cfblk18/1 -> cfblk5/2
  cfblk12/2(cfblk13) -> cfblk19/1
  cfblk19/1 -> cfblk6/1
  cfblk10/1(cfblk2) -> cfblk20/1
  cfblk20/1 -> cfblk9/1

== system sampleModel1736/cfblk86 ==
  cfblk1 : Inport
  cfblk7 : Inport  Port=2
  cfblk8 : Inport  Port=3
  cfblk9 : Inport  Port=4
  cfblk3 : Gain  Gain=[117740329.949957]
  cfblk4 : Product
  cfblk5 : Subsystem
  cfblk6 : Subsystem
  cfblk2 : Outport
  cfblk10 : Outport  Port=2
  wires:
  cfblk4/1 -> cfblk2/1
  cfblk3/1 -> cfblk6/1(cfblk1), cfblk5/6(cfblk16)
  cfblk9/1 -> cfblk5/1(cfblk1), cfblk5/5(cfblk15)
  cfblk7/1 -> cfblk6/2(cfblk14)
  cfblk1/1 -> cfblk3/1
  cfblk8/1 -> cfblk5/2(cfblk12), cfblk5/4(cfblk14)
  cfblk6/1(cfblk2) -> cfblk10/1
  cfblk6/2(cfblk15) -> cfblk5/3(cfblk13)
  cfblk5/1(cfblk2) -> cfblk4/1
  cfblk5/2(cfblk17) -> cfblk4/2

== system sampleModel1736/cfblk87 ==
  cfblk1 : Inport
  cfblk7 : Inport  Port=2
  cfblk{9..14} (6 alike) : Delay  SampleTime=1
  cfblk3 : Subsystem
  cfblk4 : Subsystem
  cfblk5 : Subsystem
  cfblk6 : Subsystem
  cfblk2 : Outport
  cfblk8 : Outport  Port=2
  wires:
  cfblk1/1 -> cfblk5/1(cfblk1), cfblk3/3(cfblk9), cfblk6/3(cfblk12)
  cfblk5/1(cfblk2) -> cfblk8/1, cfblk4/3(cfblk16)
  cfblk7/1 -> cfblk2/1, cfblk6/2(cfblk11), cfblk5/4(cfblk14)
  cfblk4/1(cfblk2) -> cfblk3/1(cfblk1), cfblk14/1
  cfblk3/3(cfblk11) -> cfblk6/1(cfblk1), cfblk6/4(cfblk13), cfblk12/1, cfblk13/1
  cfblk3/1(cfblk2) -> cfblk9/1
  cfblk9/1 -> cfblk4/1(cfblk1)
  cfblk3/2(cfblk10) -> cfblk10/1
  cfblk10/1 -> cfblk5/2(cfblk12)
  cfblk6/1(cfblk2) -> cfblk11/1
  cfblk11/1 -> cfblk3/2(cfblk8)
  cfblk12/1 -> cfblk4/2(cfblk15)
  cfblk13/1 -> cfblk5/3(cfblk13)
  cfblk14/1 -> cfblk5/5(cfblk15)

== system sampleModel1736/cfblk88 ==
  cfblk1 : Inport
  cfblk13 : Inport  Port=2
  cfblk10 : Constant  Value=[58603727.638246]  SampleTime=1
  cfblk11 : Subsystem
  cfblk12 : Subsystem
  cfblk{4,15..17} (4 alike) : Delay  SampleTime=1
  cfblk3 : simulink/Discrete/Tapped Delay  vinit=0.0  samptime=-1  NumDelays=1  DelayOrder=Oldest  includeCurrent=off
  cfblk5 : Bias  Bias=[-697996269.672310]  SaturateOnIntegerOverflow=off
  cfblk6 : Reshape
  cfblk7 : Sum  Inputs=+-
  cfblk8 : Rounding
  cfblk9 : Abs  SaturateOnIntegerOverflow=off
  cfblk2 : Outport
  cfblk14 : Outport  Port=2
  wires:
  cfblk13/1 -> cfblk2/1
  cfblk11/1(cfblk2) -> cfblk8/1
  cfblk10/1 -> cfblk12/1(cfblk1)
  cfblk12/1(cfblk2) -> cfblk4/1
  cfblk9/1 -> cfblk6/1, cfblk16/1
  cfblk7/1 -> cfblk9/1
  cfblk8/1 -> cfblk7/1
  cfblk11/2(cfblk10) -> cfblk12/2(cfblk7)
  cfblk4/1 -> cfblk14/1
  cfblk6/1 -> cfblk12/3(cfblk8)
  cfblk11/3(cfblk11) -> cfblk5/1
  cfblk5/1 -> cfblk3/1
  cfblk1/1 -> cfblk11/2(cfblk8)
  cfblk12/2(cfblk9) -> cfblk15/1
  cfblk15/1 -> cfblk7/2
  cfblk16/1 -> cfblk11/3(cfblk9)
  cfblk3/1 -> cfblk17/1
  cfblk17/1 -> cfblk11/1(cfblk1)

== system sampleModel1736/cfblk89 ==
  cfblk1 : Inport
  cfblk3 : slpidlib/PID Controller (2DOF)  Controller=PID  Form=Parallel  TimeDomain=Discrete-time  UseExternalTs=off  SampleTime=1  IntegratorMethod=Forward Euler  FilterMethod=Forward Euler  ControllerParametersSource=internal  P=1  I=1  UseKiTs=off  D=0  N=100  UseFilter=on  b=1  c=1  TunerSelectOption=Transfer Function Based (PID Tuner App)  InitialConditionSource=internal  InitialConditionForIntegrator=0  InitialConditionForFilter=0  DifferentiatorICPrevScaledInput=0  ExternalReset=none  TrackingMode=off  Kt=1  LimitOutput=off  SatLimitsSource=internal  UpperSaturationLimit=inf  LowerSaturationLimit=-inf  LinearizeAsGain=off  AntiWindupMode=none  Kb=1  POutMin=[]  POutMax=[]  IOutMin=[]  IOutMax=[]  DOutMin=[]  DOutMax=[]  NOutMin=[]  NOutMax=[]  bOutMin=[]  bOutMax=[]  cOutMin=[]  cOutMax=[]  SumOutMin=[]  SumOutMax=[]  SaturationOutMin=[]  SaturationOutMax=[]  PParamMin=[]  PParamMax=[]  IParamMin=[]  IParamMax=[]  DParamMin=[]  DParamMax=[]  NParamMin=[]  NParamMax=[]  bParamMin=[]  bParamMax=[]  cParamMin=[]  cParamMax=[]  KbParamMin=[]  KbParamMax=[]  KtParamMin=[]  KtParamMax=[]  KbOutMin=[]  KbOutMax=[]  KtOutMin=[]  KtOutMax=[]  IntegratorOutMin=[]  IntegratorOutMax=[]  FilterOutMin=[]  FilterOutMax=[]  SumI1OutMin=[]  SumI1OutMax=[]  SumI2OutMin=[]  SumI2OutMax=[]  SumI3OutMin=[]  SumI3OutMax=[]  SumI4OutMin=[]  SumI4OutMax=[]  SumDOutMin=[]  SumDOutMax=[]  Sum1OutMin=[]  Sum1OutMax=[]  Sum2OutMin=[]  Sum2OutMax=[]  Sum3OutMin=[]  Sum3OutMax=[]  DifferentiatorOutMin=[]  DifferentiatorOutMax=[]  FilterDiffOutCoefMin=[]  FilterDiffOutCoefMax=[]  ReciprocalOutMin=[]  ReciprocalOutMax=[]  SumDenOutMin=[]  SumDenOutMax=[]  SumNumOutMin=[]  SumNumOutMax=[]  DivideOutMin=[]  DivideOutMax=[]  UdiffTsProdOutMin=[]  UdiffTsProdOutMax=[]  NTsProdOutMin=[]  NTsProdOutMax=[]  UintegralTsProdOutMin=[]  UintegralTsProdOutMax=[]  UngainTsProdOutMin=[]  UngainTsProdOutMax=[]  IntegratorContinuousStateAttributes=''  IntegratorStateMustResolveToSignalObject=off  IntegratorRTWStateStorageClass=Auto  FilterContinuousStateAttributes=''  FilterStateMustResolveToSignalObject=off  FilterRTWStateStorageClass=Auto  ParallelPVariant=InternalParameters  IdealPVariant=Disabled  IVariant=InternalParameters  DVariant=InternalParameters  bVariant=InternalParameters  cVariant=InternalParameters  IntegratorVariant=Discrete  SatVariant=Disabled  AWVariant=Passthrough  PCopyVariant=Disabled  TRVariant=Disabled  FdbkBlocksVariant=Forward  IdealPFdbkVariant=Disabled  SatFdbkVariant=Disabled  DerivativeFilterVariant=ForwardEulerFilter  NVariant=InternalParameters  NCopyVariant=Disabled  FilterICVariant=InternalICsFilter  IntegratorICVariant=InternalICs  ExternalResetVariant=Disabled  TRSumVariant=Passthrough  SumFdbkVariant=Disabled  SumVariant=Sum_PID  TsampFilterVariant=InternalTs  TsampNgainVariant=Passthrough  TsampIntegralVariant=Passthrough  ExternalSaturationOutDataTypeStr=Inherit: Same as second input
      settings: SourceProductBaseCode=SL
  cfblk4 : DiscreteFir  SampleTime=1
  cfblk5 : ComplexToRealImag
  cfblk6 : Constant  Value=[-578083483.631709]  SampleTime=1
  cfblk7 : Subsystem
  cfblk8 : Delay  SampleTime=1
  cfblk2 : Outport
  wires:
  cfblk7/1(cfblk2) -> cfblk2/1
  cfblk4/1 -> cfblk7/1(cfblk1)
  cfblk6/1 -> cfblk7/2(cfblk11)
  cfblk1/1 -> cfblk5/1, cfblk3/2
  cfblk5/1 -> cfblk7/3(cfblk12)
  cfblk5/2 -> cfblk4/1
  cfblk7/2(cfblk14) -> cfblk3/1
  cfblk3/1 -> cfblk8/1
  cfblk8/1 -> cfblk7/4(cfblk13)

== system sampleModel1736/cfblk90 ==
  cfblk1 : Inport
  cfblk6 : Inport  Port=2
  cfblk7 : Inport  Port=3
  cfblk3 : Delay  DelayLengthSource=Input port  SampleTime=1
      settings: InputPortMap=u0,p1
  cfblk4 : Sum  Inputs=|++
  cfblk5 : PermuteDimensions
  cfblk2 : Outport
  wires:
  cfblk1/1 -> cfblk5/1
  cfblk6/1 -> cfblk4/1
  cfblk3/1 -> cfblk4/2
  cfblk4/1 -> cfblk2/1
  cfblk5/1 -> cfblk3/1
  cfblk7/1 -> cfblk3/2

== system sampleModel1736/cfblk91 ==
  cfblk1 : Inport
  cfblk10 : Subsystem
  cfblk{12..15} (4 alike) : Delay  SampleTime=1
  cfblk3 : DiscreteIntegrator  ICPrevOutput=DiscIntNeverNeededParam  ICPrevScaledInput=DiscIntNeverNeededParam
  cfblk4 : DiscreteZeroPole  Poles=[0 0.5]  Gain=1
  cfblk5 : simulink/Discrete/Tapped Delay  vinit=0.0  samptime=-1  NumDelays=1  DelayOrder=Oldest  includeCurrent=off
  cfblk6 : Signum
  cfblk7 : Sum  Inputs=+-
  cfblk8 : Sin  TimeSource=Use external signal  SampleTime=0
  cfblk9 : Subsystem
  cfblk2 : Outport
  cfblk11 : Outport  Port=2
  wires:
  cfblk10/1(cfblk2) -> cfblk2/1
  cfblk7/1 -> cfblk6/1, cfblk14/1
  cfblk1/1 -> cfblk9/1(cfblk1), cfblk9/4(cfblk11)
  cfblk3/1 -> cfblk11/1
  cfblk4/1 -> cfblk5/1, cfblk15/1
  cfblk8/1 -> cfblk12/1, cfblk13/1
  cfblk10/2(cfblk15) -> cfblk7/1, cfblk4/1
  cfblk9/1(cfblk2) -> cfblk10/1(cfblk1)
  cfblk5/1 -> cfblk7/2
  cfblk6/1 -> cfblk8/1
  cfblk9/2(cfblk13) -> cfblk3/1
  cfblk12/1 -> cfblk9/2(cfblk9)
  cfblk13/1 -> cfblk9/3(cfblk10)
  cfblk14/1 -> cfblk9/5(cfblk12)
  cfblk15/1 -> cfblk10/2(cfblk14)

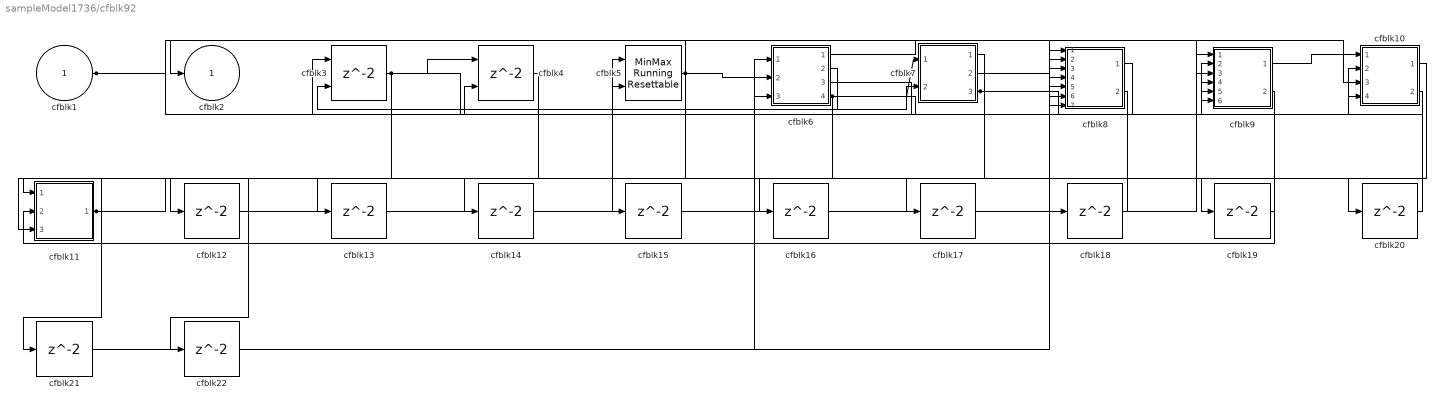
== system sampleModel1736/cfblk92 ==
  cfblk1 : Inport
  cfblk10 : Subsystem
  cfblk11 : Subsystem
  cfblk{12..22} (11 alike) : Delay  SampleTime=1
  cfblk3 : Delay  ShowEnablePort=on  SampleTime=1
      settings: InputPortMap=u0,e6
  cfblk4 : Delay  ShowEnablePort=on  SampleTime=1
      settings: InputPortMap=u0,e6
  cfblk5 : simulink/Math Operations/MinMax Running Resettable  Function=min  vinit=0.0
  cfblk6 : Subsystem
  cfblk7 : Subsystem
  cfblk8 : Subsystem
  cfblk9 : Subsystem
  cfblk2 : Outport
  wires:
  cfblk5/1 -> cfblk2/1, cfblk6/2(cfblk11), cfblk12/1
  cfblk9/1(cfblk2) -> cfblk10/1(cfblk1)
  cfblk8/1(cfblk2) -> cfblk5/1
  cfblk3/1 -> cfblk4/1, cfblk11/3(cfblk12), cfblk9/6(cfblk14), cfblk7/2(cfblk9), cfblk21/1
  cfblk11/1(cfblk2) -> cfblk15/1, cfblk16/1
  cfblk8/2(cfblk17) -> cfblk11/1(cfblk1)
  cfblk7/3(cfblk11) -> cfblk9/2(cfblk10), cfblk9/5(cfblk13), cfblk19/1, cfblk20/1
  cfblk1/1 -> cfblk8/2(cfblk11), cfblk10/3(cfblk5), cfblk10/4(cfblk6)
  cfblk9/2(cfblk15) -> cfblk11/2(cfblk11)
  cfblk10/2(cfblk7) -> cfblk4/2
  cfblk6/1(cfblk2) -> cfblk9/3(cfblk11)
  cfblk6/2(cfblk13) -> cfblk3/2
  cfblk6/3(cfblk14) -> cfblk9/4(cfblk12)
  cfblk6/4(cfblk15) -> cfblk7/1(cfblk1), cfblk10/2(cfblk4), cfblk22/1
  cfblk12/1 -> cfblk8/3(cfblk12)
  cfblk10/1(cfblk2) -> cfblk13/1
  cfblk13/1 -> cfblk5/2
  cfblk4/1 -> cfblk14/1
  cfblk14/1 -> cfblk9/1(cfblk1)
  cfblk15/1 -> cfblk6/1(cfblk1)
  cfblk16/1 -> cfblk8/6(cfblk15)
  cfblk7/1(cfblk2) -> cfblk17/1
  cfblk17/1 -> cfblk8/1(cfblk1)
  cfblk7/2(cfblk10) -> cfblk18/1
  cfblk18/1 -> cfblk3/1
  cfblk19/1 -> cfblk8/4(cfblk13)
  cfblk20/1 -> cfblk8/5(cfblk14)
  cfblk21/1 -> cfblk6/3(cfblk12)
  cfblk22/1 -> cfblk8/7(cfblk16)

== system sampleModel1736/cfblk93 ==
  cfblk1 : Inport
  cfblk11 : Inport  Port=2
  cfblk10 : Subsystem
  cfblk13 : Delay  SampleTime=1
  cfblk14 : Delay  SampleTime=1
  cfblk3 : simulink/Discrete/Difference  ICPrevInput=0.0  OutMin=[]  OutMax=[]  OutDataTypeStr=Inherit: Inherit via back propagation  OutDataType=fixdt(1, 16)  OutScaling=2^-10  DoSatur=off
  cfblk4 : Delay  SampleTime=1
  cfblk5 : Delay  DelayLengthSource=Input port  SampleTime=1
      settings: InputPortMap=u0,p1
  cfblk6 : Reshape
  cfblk7 : simulink/Math Operations/Slider Gain  gain=1  low=0  high=2
  cfblk8 : Constant  Value=[-550157555.054569]  SampleTime=1
  cfblk9 : Subsystem
  cfblk2 : Outport
  cfblk12 : Outport  Port=2
  wires:
  cfblk7/1 -> cfblk10/1(cfblk1)
  cfblk9/1(cfblk2) -> cfblk10/2(cfblk10)
  cfblk5/1 -> cfblk7/1
  cfblk1/1 -> cfblk9/1(cfblk1)
  cfblk10/1(cfblk2) -> cfblk4/1
  cfblk8/1 -> cfblk12/1
  cfblk3/1 -> cfblk5/1
  cfblk11/1 -> cfblk5/2
  cfblk9/2(cfblk16) -> cfblk3/1
  cfblk6/1 -> cfblk13/1, cfblk14/1
  cfblk10/2(cfblk11) -> cfblk6/1
  cfblk4/1 -> cfblk2/1
  cfblk13/1 -> cfblk9/2(cfblk14)
  cfblk14/1 -> cfblk9/3(cfblk15)

== system sampleModel1736/cfblk94 ==
  cfblk1 : Inport
  cfblk{8..14} (7 alike) : Delay  SampleTime=1
  cfblk3 : Constant  Value=[-18267472.809538]  SampleTime=1
  cfblk4 : Subsystem
  cfblk5 : Subsystem
  cfblk6 : Subsystem
  cfblk2 : Outport
  cfblk7 : Outport  Port=2
  wires:
  cfblk1/1 -> cfblk5/1(cfblk1), cfblk6/3(cfblk9)
  cfblk3/1 -> cfblk7/1, cfblk6/5(cfblk11)
  cfblk5/1(cfblk2) -> cfblk6/1(cfblk1)
  cfblk6/3(cfblk13) -> cfblk4/2(cfblk13), cfblk10/1
  cfblk5/2(cfblk16) -> cfblk4/1(cfblk1), cfblk4/3(cfblk14), cfblk4/4(cfblk15), cfblk6/4(cfblk10)
  cfblk4/3(cfblk17) -> cfblk2/1, cfblk13/1, cfblk14/1
  cfblk6/1(cfblk2) -> cfblk8/1
  cfblk8/1 -> cfblk5/3(cfblk11)
  cfblk6/2(cfblk12) -> cfblk9/1
  cfblk9/1 -> cfblk5/4(cfblk12)
  cfblk10/1 -> cfblk5/5(cfblk13)
  cfblk4/1(cfblk2) -> cfblk11/1
  cfblk11/1 -> cfblk5/2(cfblk10)
  cfblk4/2(cfblk16) -> cfblk12/1
  cfblk12/1 -> cfblk5/6(cfblk14)
  cfblk13/1 -> cfblk5/7(cfblk15)
  cfblk14/1 -> cfblk6/2(cfblk8)

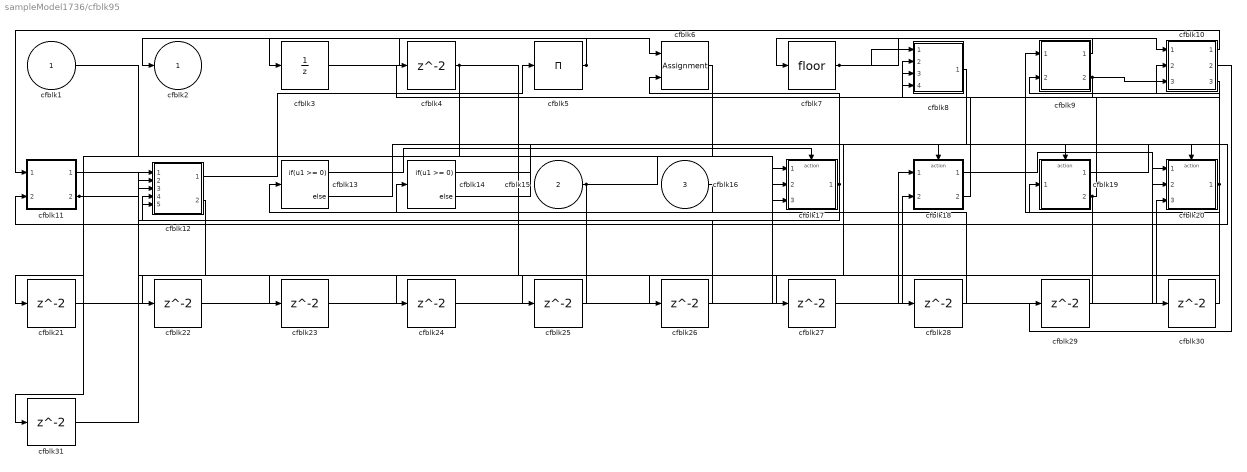
== system sampleModel1736/cfblk95 ==
  cfblk1 : Inport
  cfblk15 : Inport  Port=2
  cfblk16 : Inport  Port=3
  cfblk10 : Subsystem
  cfblk11 : Subsystem
  cfblk12 : Subsystem
  cfblk13 : If  IfExpression=u1 >= 0  SampleTime=1
  cfblk14 : If  IfExpression=u1 >= 0  SampleTime=1
  cfblk17 : Subsystem  TreatAsAtomicUnit=on
  cfblk18 : Subsystem  TreatAsAtomicUnit=on
  cfblk19 : Subsystem  TreatAsAtomicUnit=on
  cfblk20 : Subsystem  TreatAsAtomicUnit=on
  cfblk{4,21..31} (12 alike) : Delay  SampleTime=1
  cfblk3 : UnitDelay  HasFrameUpgradeWarning=on
  cfblk5 : Product  Inputs=*
  cfblk6 : Assignment  DiagnosticForDimensions=Warning  IndexOptions=Index vector (dialog)  Indices=1  OutputSizes=1
  cfblk7 : Rounding
  cfblk8 : Subsystem
  cfblk9 : Subsystem
  cfblk2 : Outport
  wires:
  cfblk9/1(cfblk2) -> cfblk7/1
  cfblk5/1 -> cfblk2/1, cfblk3/1
  cfblk12/1(cfblk2) -> cfblk5/1
  cfblk16/1 -> cfblk13/1
  cfblk20/1(cfblk2) -> cfblk9/2(cfblk11), cfblk10/2(cfblk14), cfblk28/1
  cfblk3/1 -> cfblk6/1
  cfblk7/1 -> cfblk8/1(cfblk1), cfblk10/1(cfblk1)
  cfblk15/1 -> cfblk17/2(cfblk10), cfblk12/4(cfblk11)
  cfblk10/1(cfblk2) -> cfblk11/1(cfblk1)
  cfblk17/1(cfblk2) -> cfblk6/2, cfblk12/5(cfblk12)
  cfblk11/2(cfblk10) -> cfblk24/1, cfblk25/1
  cfblk1/1 -> cfblk17/3(cfblk11)
  cfblk4/1 -> cfblk30/1, cfblk31/1
  cfblk19/1(cfblk2) -> cfblk11/2(cfblk9)
  cfblk18/1(cfblk2) -> cfblk20/2(cfblk10)
  cfblk9/2(cfblk12) -> cfblk4/1, cfblk10/3(cfblk15)
  cfblk19/2(cfblk10) -> cfblk8/4(cfblk14), cfblk26/1
  cfblk10/3(cfblk17) -> cfblk8/2(cfblk12)
  cfblk18/2(cfblk8) -> cfblk8/3(cfblk13)
  cfblk13/1 -> cfblk17/Action
  cfblk13/2 -> cfblk18/Action
  cfblk14/1 -> cfblk19/Action
  cfblk14/2 -> cfblk20/Action
  cfblk6/1 -> cfblk21/1
  cfblk21/1 -> cfblk17/1(cfblk1)
  cfblk12/2(cfblk13) -> cfblk22/1
  cfblk22/1 -> cfblk18/1(cfblk1)
  cfblk11/1(cfblk2) -> cfblk23/1
  cfblk23/1 -> cfblk18/2(cfblk7)
  cfblk24/1 -> cfblk20/1(cfblk1)
  cfblk25/1 -> cfblk12/3(cfblk10)
  cfblk26/1 -> cfblk12/1(cfblk1)
  cfblk8/1(cfblk2) -> cfblk27/1
  cfblk27/1 -> cfblk20/3(cfblk11)
  cfblk28/1 -> cfblk14/1
  cfblk10/2(cfblk16) -> cfblk29/1
  cfblk29/1 -> cfblk9/1(cfblk1)
  cfblk30/1 -> cfblk19/1(cfblk1)
  cfblk31/1 -> cfblk12/2(cfblk9)

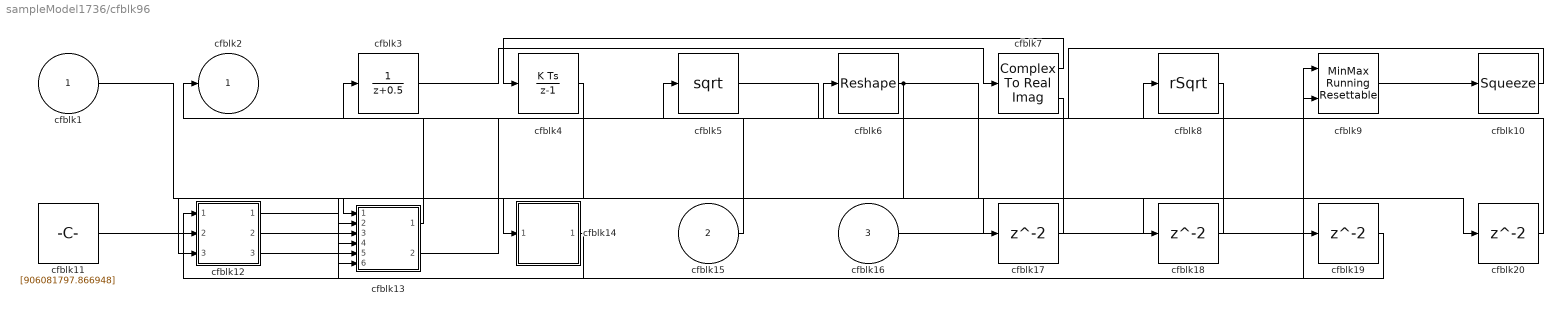
== system sampleModel1736/cfblk96 ==
  cfblk1 : Inport
  cfblk15 : Inport  Port=2
  cfblk16 : Inport  Port=3
  cfblk10 : Squeeze
  cfblk11 : Constant  Value=[906081797.866948]  SampleTime=1
  cfblk12 : Subsystem
  cfblk13 : Subsystem
  cfblk14 : Subsystem
  cfblk{17..20} (4 alike) : Delay  SampleTime=1
  cfblk3 : DiscreteTransferFcn  SampleTime=1
  cfblk4 : DiscreteIntegrator  ICPrevOutput=DiscIntNeverNeededParam  ICPrevScaledInput=DiscIntNeverNeededParam
  cfblk5 : Sqrt
  cfblk6 : Reshape
  cfblk7 : ComplexToRealImag
  cfblk8 : Sqrt  Operator=rSqrt  AlgorithmType=Newton-Raphson
  cfblk9 : simulink/Math Operations/MinMax Running Resettable  Function=min  vinit=0.0
  cfblk2 : Outport
  wires:
  cfblk9/1 -> cfblk10/1
  cfblk6/1 -> cfblk13/6(cfblk13), cfblk20/1
  cfblk13/1(cfblk2) -> cfblk2/1
  cfblk7/1 -> cfblk4/1
  cfblk16/1 -> cfblk9/1
  cfblk10/1 -> cfblk6/1
  cfblk1/1 -> cfblk13/1(cfblk1)
  cfblk14/1(cfblk2) -> cfblk12/1(cfblk1)
  cfblk4/1 -> cfblk14/1(cfblk1)
  cfblk8/1 -> cfblk12/2(cfblk12)
  cfblk3/1 -> cfblk7/1
  cfblk11/1 -> cfblk12/3(cfblk13)
  cfblk13/2(cfblk14) -> cfblk8/1
  cfblk7/2 -> cfblk13/3(cfblk10)
  cfblk5/1 -> cfblk9/2
  cfblk15/1 -> cfblk3/1
  cfblk12/1(cfblk2) -> cfblk17/1
  cfblk17/1 -> cfblk13/2(cfblk9)
  cfblk12/2(cfblk14) -> cfblk18/1
  cfblk18/1 -> cfblk13/4(cfblk11)
  cfblk12/3(cfblk15) -> cfblk19/1
  cfblk19/1 -> cfblk13/5(cfblk12)
  cfblk20/1 -> cfblk5/1
